simulink library "Simscape_Gates_Lib"  (R2023a)
settings: Solver=VariableStepAuto  StartTime=0.0  StopTime=10.0  RelTol=1e-3
libraries: ee_lib x80
(part 2 of 2)

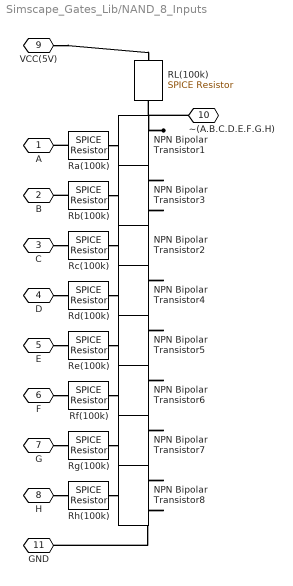
== system Simscape_Gates_Lib/NAND_8_Inputs ==
  NPN Bipolar Transistor{1..8} (8 alike) : ee_lib/Semiconductors & Converters/NPN Bipolar Transistor  parameterization=1  BF=100  IS=1e-14 A  VAF=200 V  hfe=100  hoe=5e-5 1/Ohm  Ic_h=1 mA  Vce_h=5 V  V1=0.55 V  I1=0.5 mA  BR=1  Tmeas=25 degC  RC=0.01 Ohm  RE=1e-4 Ohm  RB=1 Ohm  C_BC=5 pF  C_BE=5 pF  TF=0 us  TR=0 us  prmDatasheet=1  prmEquCoeff=1  hfe_T2=125  XTB=0  V1_T2=0.45 V  I1_T2=0.5 mA  Tmeas2=125 degC  EG=1.11 eV  XTI=3  TdeviceDatasheet=25 degC  TdeviceEquCoeff=25 degC  ec=1  ib_specify=off  ib_priority=None  ib=0 A  ib_nominal_specify=off  ib_nominal_unit=A  ib_nominal_value=1  ic_specify=off  ic_priority=None  ic=0 A  ic_nominal_specify=off  ic_nominal_unit=A  ic_nominal_value=1  vce_specify=off  vce_priority=None  vce=0 V  vce_nominal_specify=off  vce_nominal_unit=V  vce_nominal_value=1  vbe_specify=off  vbe_priority=None  vbe=0 V  vbe_nominal_specify=off  vbe_nominal_unit=V  vbe_nominal_value=1  v_capacitor_bc_specify=off  v_capacitor_bc_priority=High  v_capacitor_bc=0 V  v_capacitor_bc_nominal_specify=off  v_capacitor_bc_nominal_unit=V  v_capacitor_bc_nominal_value=1  v_capacitor_be_specify=off  v_capacitor_be_priority=High  v_capacitor_be=0 V  v_capacitor_be_nominal_specify=off  v_capacitor_be_nominal_unit=V  v_capacitor_be_nominal_value=1  thermal_network_parameterization=ee.enum.thermalNetworkTopology.junctionCase  Rth=[0, 10] K/W  Rth_Cauer=[1, 3, 10] K/W  Rth_Foster=[4, 6] K/W  thermal_mass_parameterization=ee.enum.thermalNetwork.timeconstant  thermal_mass=[0, 1] J/K  thermal_mass_Cauer=[.1, .3, 1] J/K  thermal_mass_Foster=[1.5, 3] J/K  thermal_time_constant=[0, 10] s  thermal_time_constant_Cauer=[1, 3, 10] s  thermal_time_constant_Foster=[6, 18] s  thermal_mass_initial_temperatures=[25, 25] degC  thermal_mass_initial_temperatures_Cauer=[25, 25, 25] degC  Tvec_initial_Foster=[25, 25, 25, 25] degC
  RL(100k) : ee_lib/Additional Components/SPICE Passives/SPICE Resistor  SCALE=1.0  R_param=1  R=100 kOhm  RSH=0 Ohm  LENGTH=1e-6 m  WIDTH=1e-6 m  NARROW=0 m  T_param=1  TC1=0 1/K  TC2=0 1/K^2  TOFFSET=0 K  TFIXED=300.15 K  TMEAS=300.15 K
      settings: InternalSimscapePortConfiguration="{\"Bottom\":[],\"Left\":[{\"id\":\"p\",\"label\":\"\",\"type\":\"foundation.electrical.electrical\"}],\"Right\":[{\"id\":\"n\",\"label\":\"\",\"type\":\"foundation.electrical.electrical\"}],\"Top\":[]}"
  Ra(100k) : ee_lib/Additional Components/SPICE Passives/SPICE Resistor  SCALE=1.0  R_param=1  R=100 kOhm  RSH=0 Ohm  LENGTH=1e-6 m  WIDTH=1e-6 m  NARROW=0 m  T_param=1  TC1=0 1/K  TC2=0 1/K^2  TOFFSET=0 K  TFIXED=300.15 K  TMEAS=300.15 K
      settings: InternalSimscapePortConfiguration="{\"Bottom\":[],\"Left\":[{\"id\":\"p\",\"label\":\"\",\"type\":\"foundation.electrical.electrical\"}],\"Right\":[{\"id\":\"n\",\"label\":\"\",\"type\":\"foundation.electrical.electrical\"}],\"Top\":[]}"
  Rb(100k) : ee_lib/Additional Components/SPICE Passives/SPICE Resistor  SCALE=1.0  R_param=1  R=100 kOhm  RSH=0 Ohm  LENGTH=1e-6 m  WIDTH=1e-6 m  NARROW=0 m  T_param=1  TC1=0 1/K  TC2=0 1/K^2  TOFFSET=0 K  TFIXED=300.15 K  TMEAS=300.15 K
      settings: InternalSimscapePortConfiguration="{\"Bottom\":[],\"Left\":[{\"id\":\"p\",\"label\":\"\",\"type\":\"foundation.electrical.electrical\"}],\"Right\":[{\"id\":\"n\",\"label\":\"\",\"type\":\"foundation.electrical.electrical\"}],\"Top\":[]}"
  Rc(100k) : ee_lib/Additional Components/SPICE Passives/SPICE Resistor  SCALE=1.0  R_param=1  R=100 kOhm  RSH=0 Ohm  LENGTH=1e-6 m  WIDTH=1e-6 m  NARROW=0 m  T_param=1  TC1=0 1/K  TC2=0 1/K^2  TOFFSET=0 K  TFIXED=300.15 K  TMEAS=300.15 K
      settings: InternalSimscapePortConfiguration="{\"Bottom\":[],\"Left\":[{\"id\":\"p\",\"label\":\"\",\"type\":\"foundation.electrical.electrical\"}],\"Right\":[{\"id\":\"n\",\"label\":\"\",\"type\":\"foundation.electrical.electrical\"}],\"Top\":[]}"
  Rd(100k) : ee_lib/Additional Components/SPICE Passives/SPICE Resistor  SCALE=1.0  R_param=1  R=100 kOhm  RSH=0 Ohm  LENGTH=1e-6 m  WIDTH=1e-6 m  NARROW=0 m  T_param=1  TC1=0 1/K  TC2=0 1/K^2  TOFFSET=0 K  TFIXED=300.15 K  TMEAS=300.15 K
      settings: InternalSimscapePortConfiguration="{\"Bottom\":[],\"Left\":[{\"id\":\"p\",\"label\":\"\",\"type\":\"foundation.electrical.electrical\"}],\"Right\":[{\"id\":\"n\",\"label\":\"\",\"type\":\"foundation.electrical.electrical\"}],\"Top\":[]}"
  Re(100k) : ee_lib/Additional Components/SPICE Passives/SPICE Resistor  SCALE=1.0  R_param=1  R=100 kOhm  RSH=0 Ohm  LENGTH=1e-6 m  WIDTH=1e-6 m  NARROW=0 m  T_param=1  TC1=0 1/K  TC2=0 1/K^2  TOFFSET=0 K  TFIXED=300.15 K  TMEAS=300.15 K
      settings: InternalSimscapePortConfiguration="{\"Bottom\":[],\"Left\":[{\"id\":\"p\",\"label\":\"\",\"type\":\"foundation.electrical.electrical\"}],\"Right\":[{\"id\":\"n\",\"label\":\"\",\"type\":\"foundation.electrical.electrical\"}],\"Top\":[]}"
  Rf(100k) : ee_lib/Additional Components/SPICE Passives/SPICE Resistor  SCALE=1.0  R_param=1  R=100 kOhm  RSH=0 Ohm  LENGTH=1e-6 m  WIDTH=1e-6 m  NARROW=0 m  T_param=1  TC1=0 1/K  TC2=0 1/K^2  TOFFSET=0 K  TFIXED=300.15 K  TMEAS=300.15 K
      settings: InternalSimscapePortConfiguration="{\"Bottom\":[],\"Left\":[{\"id\":\"p\",\"label\":\"\",\"type\":\"foundation.electrical.electrical\"}],\"Right\":[{\"id\":\"n\",\"label\":\"\",\"type\":\"foundation.electrical.electrical\"}],\"Top\":[]}"
  Rg(100k) : ee_lib/Additional Components/SPICE Passives/SPICE Resistor  SCALE=1.0  R_param=1  R=100 kOhm  RSH=0 Ohm  LENGTH=1e-6 m  WIDTH=1e-6 m  NARROW=0 m  T_param=1  TC1=0 1/K  TC2=0 1/K^2  TOFFSET=0 K  TFIXED=300.15 K  TMEAS=300.15 K
      settings: InternalSimscapePortConfiguration="{\"Bottom\":[],\"Left\":[{\"id\":\"p\",\"label\":\"\",\"type\":\"foundation.electrical.electrical\"}],\"Right\":[{\"id\":\"n\",\"label\":\"\",\"type\":\"foundation.electrical.electrical\"}],\"Top\":[]}"
  Rh(100k) : ee_lib/Additional Components/SPICE Passives/SPICE Resistor  SCALE=1.0  R_param=1  R=100 kOhm  RSH=0 Ohm  LENGTH=1e-6 m  WIDTH=1e-6 m  NARROW=0 m  T_param=1  TC1=0 1/K  TC2=0 1/K^2  TOFFSET=0 K  TFIXED=300.15 K  TMEAS=300.15 K
      settings: InternalSimscapePortConfiguration="{\"Bottom\":[],\"Left\":[{\"id\":\"p\",\"label\":\"\",\"type\":\"foundation.electrical.electrical\"}],\"Right\":[{\"id\":\"n\",\"label\":\"\",\"type\":\"foundation.electrical.electrical\"}],\"Top\":[]}"
  A : PMIOPort  Side=Left
  B : PMIOPort  Port=2  Side=Left
  C : PMIOPort  Port=3  Side=Left
  D : PMIOPort  Port=4  Side=Left
  E : PMIOPort  Port=5  Side=Left
  F : PMIOPort  Port=6  Side=Left
  G : PMIOPort  Port=7  Side=Left
  H : PMIOPort  Port=8  Side=Left
  VCC(5V) : PMIOPort  Port=9  Side=Left
  ~(A.B.C.D.E.F.G.H) : PMIOPort  Port=10  Side=Right
  GND : PMIOPort  Port=11  Side=Right
  connections:
  NPN Bipolar Transistor1/RConn1 -- ~(A.B.C.D.E.F.G.H)/RConn1 -- RL(100k)/LConn1
  Rf(100k)/LConn1 -- NPN Bipolar Transistor6/LConn1
  NPN Bipolar Transistor8/RConn2 -- GND/RConn1
  Ra(100k)/LConn1 -- NPN Bipolar Transistor1/LConn1
  Rg(100k)/LConn1 -- NPN Bipolar Transistor7/LConn1
  Re(100k)/LConn1 -- NPN Bipolar Transistor5/LConn1
  H/RConn1 -- Rh(100k)/RConn1
  Rh(100k)/LConn1 -- NPN Bipolar Transistor8/LConn1
  D/RConn1 -- Rd(100k)/RConn1
  F/RConn1 -- Rf(100k)/RConn1
  NPN Bipolar Transistor3/RConn1 -- NPN Bipolar Transistor1/RConn2
  NPN Bipolar Transistor5/RConn1 -- NPN Bipolar Transistor4/RConn2
  NPN Bipolar Transistor4/RConn1 -- NPN Bipolar Transistor2/RConn2
  Rd(100k)/LConn1 -- NPN Bipolar Transistor4/LConn1
  NPN Bipolar Transistor6/RConn1 -- NPN Bipolar Transistor5/RConn2
  NPN Bipolar Transistor7/RConn1 -- NPN Bipolar Transistor6/RConn2
  E/RConn1 -- Re(100k)/RConn1
  VCC(5V)/RConn1 -- RL(100k)/RConn1
  Rb(100k)/RConn1 -- B/RConn1
  Ra(100k)/RConn1 -- A/RConn1
  NPN Bipolar Transistor3/RConn2 -- NPN Bipolar Transistor2/RConn1
  NPN Bipolar Transistor8/RConn1 -- NPN Bipolar Transistor7/RConn2
  Rc(100k)/LConn1 -- NPN Bipolar Transistor2/LConn1
  C/RConn1 -- Rc(100k)/RConn1
  Rb(100k)/LConn1 -- NPN Bipolar Transistor3/LConn1
  G/RConn1 -- Rg(100k)/RConn1

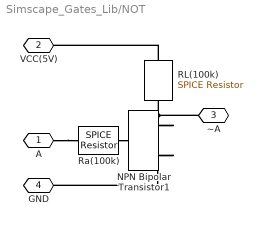
== system Simscape_Gates_Lib/NOT ==
  NPN Bipolar Transistor1 : ee_lib/Semiconductors & Converters/NPN Bipolar Transistor  parameterization=1  BF=100  IS=1e-14 A  VAF=200 V  hfe=100  hoe=5e-5 1/Ohm  Ic_h=1 mA  Vce_h=5 V  V1=0.55 V  I1=0.5 mA  BR=1  Tmeas=25 degC  RC=0.01 Ohm  RE=1e-4 Ohm  RB=1 Ohm  C_BC=5 pF  C_BE=5 pF  TF=0 us  TR=0 us  prmDatasheet=1  prmEquCoeff=1  hfe_T2=125  XTB=0  V1_T2=0.45 V  I1_T2=0.5 mA  Tmeas2=125 degC  EG=1.11 eV  XTI=3  TdeviceDatasheet=25 degC  TdeviceEquCoeff=25 degC  ec=1  ib_specify=off  ib_priority=None  ib=0 A  ib_nominal_specify=off  ib_nominal_unit=A  ib_nominal_value=1  ic_specify=off  ic_priority=None  ic=0 A  ic_nominal_specify=off  ic_nominal_unit=A  ic_nominal_value=1  vce_specify=off  vce_priority=None  vce=0 V  vce_nominal_specify=off  vce_nominal_unit=V  vce_nominal_value=1  vbe_specify=off  vbe_priority=None  vbe=0 V  vbe_nominal_specify=off  vbe_nominal_unit=V  vbe_nominal_value=1  v_capacitor_bc_specify=off  v_capacitor_bc_priority=High  v_capacitor_bc=0 V  v_capacitor_bc_nominal_specify=off  v_capacitor_bc_nominal_unit=V  v_capacitor_bc_nominal_value=1  v_capacitor_be_specify=off  v_capacitor_be_priority=High  v_capacitor_be=0 V  v_capacitor_be_nominal_specify=off  v_capacitor_be_nominal_unit=V  v_capacitor_be_nominal_value=1  thermal_network_parameterization=ee.enum.thermalNetworkTopology.junctionCase  Rth=[0, 10] K/W  Rth_Cauer=[1, 3, 10] K/W  Rth_Foster=[4, 6] K/W  thermal_mass_parameterization=ee.enum.thermalNetwork.timeconstant  thermal_mass=[0, 1] J/K  thermal_mass_Cauer=[.1, .3, 1] J/K  thermal_mass_Foster=[1.5, 3] J/K  thermal_time_constant=[0, 10] s  thermal_time_constant_Cauer=[1, 3, 10] s  thermal_time_constant_Foster=[6, 18] s  thermal_mass_initial_temperatures=[25, 25] degC  thermal_mass_initial_temperatures_Cauer=[25, 25, 25] degC  Tvec_initial_Foster=[25, 25, 25, 25] degC
  RL(100k) : ee_lib/Additional Components/SPICE Passives/SPICE Resistor  SCALE=1.0  R_param=1  R=100 kOhm  RSH=0 Ohm  LENGTH=1e-6 m  WIDTH=1e-6 m  NARROW=0 m  T_param=1  TC1=0 1/K  TC2=0 1/K^2  TOFFSET=0 K  TFIXED=300.15 K  TMEAS=300.15 K
      settings: InternalSimscapePortConfiguration="{\"Bottom\":[],\"Left\":[{\"id\":\"p\",\"label\":\"\",\"type\":\"foundation.electrical.electrical\"}],\"Right\":[{\"id\":\"n\",\"label\":\"\",\"type\":\"foundation.electrical.electrical\"}],\"Top\":[]}"
  Ra(100k) : ee_lib/Additional Components/SPICE Passives/SPICE Resistor  SCALE=1.0  R_param=1  R=100 kOhm  RSH=0 Ohm  LENGTH=1e-6 m  WIDTH=1e-6 m  NARROW=0 m  T_param=1  TC1=0 1/K  TC2=0 1/K^2  TOFFSET=0 K  TFIXED=300.15 K  TMEAS=300.15 K
      settings: InternalSimscapePortConfiguration="{\"Bottom\":[],\"Left\":[{\"id\":\"p\",\"label\":\"\",\"type\":\"foundation.electrical.electrical\"}],\"Right\":[{\"id\":\"n\",\"label\":\"\",\"type\":\"foundation.electrical.electrical\"}],\"Top\":[]}"
  A : PMIOPort  Side=Left
  VCC(5V) : PMIOPort  Port=2  Side=Left
  ~A : PMIOPort  Port=3  Side=Right
  GND : PMIOPort  Port=4  Side=Right
  connections:
  Ra(100k)/LConn1 -- NPN Bipolar Transistor1/LConn1
  NPN Bipolar Transistor1/RConn2 -- GND/RConn1
  RL(100k)/RConn1 -- NPN Bipolar Transistor1/RConn1 -- ~A/RConn1
  A/RConn1 -- Ra(100k)/RConn1
  RL(100k)/LConn1 -- VCC(5V)/RConn1
